simulink model "sim_instalacja_podlogowa_regulacja_pogodowa"  (R2021b)
settings: Solver=VariableStepAuto  StartTime=0.0  StopTime=10.0  MaxStep=10  RelTol=1e-3
undefined symbols (not defined in the file): ap_bojlera, az, az_bojlera, bp_bojlera, bz, bz_bojlera, cpw, Cvcwu, Cvgp, Cvk, Cvp, Cvr, Cvs, Cvw, delay, dpoN, dqt, dqtb, dqtb2, dRz_b, dRz_p, dTcwu, dTzew, fmbN, Kcp1, Kcp2, Kcr, Kcs, Kcw, ki_main, ki_zaw_bojler, ki_zaw_podloga, kp_main, kp_zaw_bojler, kp_zaw_podloga, qtb2N, qtbN, qtN, Rb, Rk, Rp, RzN, skok_czas, skok_czas0, skok_czas2, Tcwu0, TcwuN, Tgp0, TkpN, Tkz0, TkzN, Tp0, Trp0, TrpN, Ts0, Tset_cwu, Twew0, TwewK, Tzadana0, TzewN ... (+1)
libraries: slpidlib x3, simulink x1
settings Model: Creator=adams  LastModifiedBy=adams

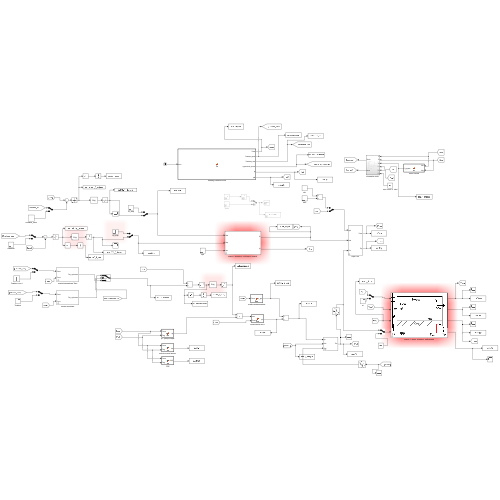
[thumbnail: Simulink's stored preview of the top-level diagram]
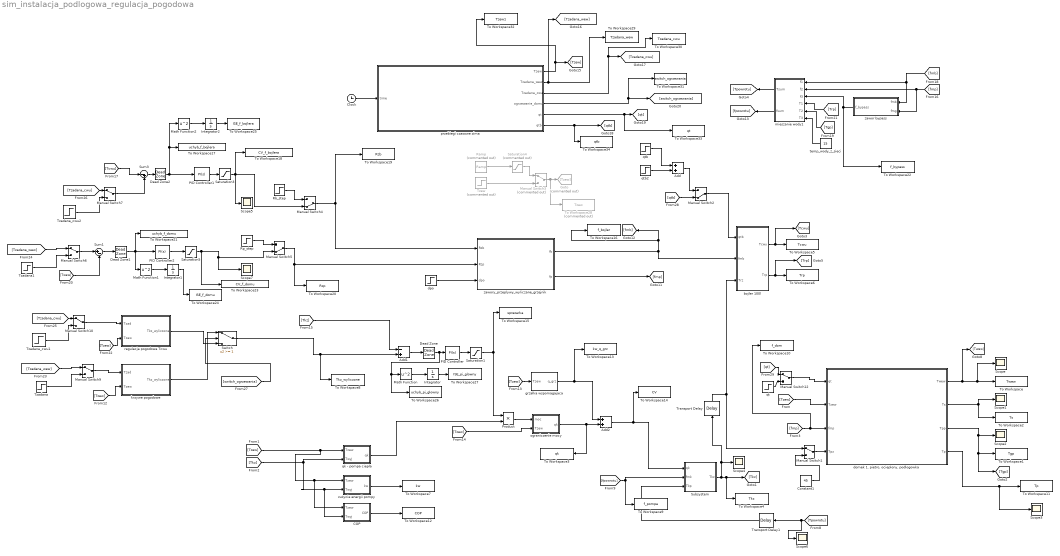
== system sim_instalacja_podlogowa_regulacja_pogodowa ==
  Add : Sum
  Add1 : Sum  Inputs=-+
  Add2 : Sum
  COP : MATLAB Function  TreatAsAtomicUnit=on
  Clock : Clock
  Constant1 : Constant  Value=45
  Dead Zone : DeadZone  LowerValue=-0.15  UpperValue=0.15  SaturateOnIntegerOverflow=on
  Dead Zone1 : DeadZone  LowerValue=-0.55  UpperValue=0.55  SaturateOnIntegerOverflow=on
  Dead Zone2 : DeadZone  LowerValue=-0.35  UpperValue=0.35  SaturateOnIntegerOverflow=on
  Goto : Goto  Commented=on  GotoTag=Tzew
  Integrator : Integrator
  Integrator1 : Integrator
  Integrator2 : Integrator
  Manual Switch{1,6..7,9..10,12} (6 alike) : ManualSwitch
  Manual Switch2 : ManualSwitch  CurrentSetting=0
  Manual Switch3 : ManualSwitch  Commented=on
  Manual Switch4 : ManualSwitch  CurrentSetting=0
  Manual Switch5 : ManualSwitch  CurrentSetting=0
  Math Function : Math  Operator=square  SaturateOnIntegerOverflow=on
  Math Function1 : Math  Operator=square  SaturateOnIntegerOverflow=on
  Math Function2 : Math  Operator=square  SaturateOnIntegerOverflow=on
  PID Controller : slpidlib/PID Controller  Controller=PI  Form=Parallel  TimeDomain=Continuous-time  UseExternalTs=off  SampleTime=-1  IntegratorMethod=Forward Euler  FilterMethod=Forward Euler  ControllerParametersSource=internal  P=kp_main  I=ki_main  D=0  UseFilter=on  N=100  TunerSelectOption=Transfer Function Based (PID Tuner App)  InitialConditionSource=internal  InitialConditionForIntegrator=1  InitialConditionForFilter=0  DifferentiatorICPrevScaledInput=0  ExternalReset=none  TrackingMode=off  Kt=1  LimitOutput=off  SatLimitsSource=internal  UpperSaturationLimit=inf  LowerSaturationLimit=-inf  LinearizeAsGain=on  AntiWindupMode=none  Kb=1  POutMin=[]  POutMax=[]  IOutMin=[]  IOutMax=[]  DOutMin=[]  DOutMax=[]  NOutMin=[]  NOutMax=[]  SumOutMin=[]  SumOutMax=[]  SaturationOutMin=[]  SaturationOutMax=[]  PParamMin=[]  PParamMax=[]  IParamMin=[]  IParamMax=[]  DParamMin=[]  DParamMax=[]  NParamMin=[]  NParamMax=[]  KbParamMin=[]  KbParamMax=[]  KtParamMin=[]  KtParamMax=[]  KbOutMin=[]  KbOutMax=[]  KtOutMin=[]  KtOutMax=[]  IntegratorOutMin=[]  IntegratorOutMax=[]  FilterOutMin=[]  FilterOutMax=[]  SumI1OutMin=[]  SumI1OutMax=[]  SumI2OutMin=[]  SumI2OutMax=[]  SumI3OutMin=[]  SumI3OutMax=[]  SumI4OutMin=[]  SumI4OutMax=[]  SumDOutMin=[]  SumDOutMax=[]  DifferentiatorOutMin=[]  DifferentiatorOutMax=[]  FilterDiffOutCoefMin=[]  FilterDiffOutCoefMax=[]  ReciprocalOutMin=[]  ReciprocalOutMax=[]  SumDenOutMin=[]  SumDenOutMax=[]  SumNumOutMin=[]  SumNumOutMax=[]  DivideOutMin=[]  DivideOutMax=[]  UdiffTsProdOutMin=[]  UdiffTsProdOutMax=[]  NTsProdOutMin=[]  NTsProdOutMax=[]  UintegralTsProdOutMin=[]  UintegralTsProdOutMax=[]  UngainTsProdOutMin=[]  UngainTsProdOutMax=[]  FilterDenConstantOutDataTypeStr=Inherit: Inherit via back propagation  FilterDenConstantOutMin=[]  FilterDenConstantOutMax=[]  PCopyOutDataTypeStr=Inherit: Inherit via back propagation  PCopyOutMin=[]  PCopyOutMax=[]  NCopyOutDataTypeStr=Inherit: Inherit via back propagation  NCopyOutMin=[]  NCopyOutMax=[]  IntegratorContinuousStateAttributes=''  IntegratorStateMustResolveToSignalObject=off  IntegratorRTWStateStorageClass=Auto  FilterContinuousStateAttributes=''  FilterStateMustResolveToSignalObject=off  FilterRTWStateStorageClass=Auto  ParallelPVariant=InternalParameters  IdealPVariant=Disabled  IVariant=InternalParameters  DVariant=Disabled  IntegratorVariant=Continuous  SatVariant=Disabled  AWVariant=Passthrough  PCopyVariant=Disabled  TRVariant=Disabled  FdbkBlocksVariant=Forward  IdealPFdbkVariant=Disabled  SatFdbkVariant=Disabled  DerivativeFilterVariant=Disabled  NVariant=Disabled  NCopyVariant=Disabled_SignalSpec  FilterICVariant=Disabled  IntegratorICVariant=InternalICs  ExternalResetVariant=Disabled  TRSumVariant=Passthrough  SumFdbkVariant=Disabled  SumVariant=Sum_PI  TsampFilterVariant=InternalTs  TsampNgainVariant=Passthrough  TsampIntegralVariant=Passthrough  ExternalSaturationOutDataTypeStr=Inherit: Same as second input
  PID Controller1 : slpidlib/PID Controller  Controller=PI  Form=Parallel  TimeDomain=Continuous-time  UseExternalTs=off  SampleTime=-1  IntegratorMethod=Forward Euler  FilterMethod=Forward Euler  ControllerParametersSource=internal  P=kp_zaw_bojler  I=ki_zaw_bojler  D=0  UseFilter=on  N=100  TunerSelectOption=Transfer Function Based (PID Tuner App)  InitialConditionSource=internal  InitialConditionForIntegrator=0  InitialConditionForFilter=0  DifferentiatorICPrevScaledInput=0  ExternalReset=none  TrackingMode=off  Kt=1  LimitOutput=off  SatLimitsSource=internal  UpperSaturationLimit=inf  LowerSaturationLimit=-inf  LinearizeAsGain=on  AntiWindupMode=none  Kb=1  POutMin=[]  POutMax=[]  IOutMin=[]  IOutMax=[]  DOutMin=[]  DOutMax=[]  NOutMin=[]  NOutMax=[]  SumOutMin=[]  SumOutMax=[]  SaturationOutMin=[]  SaturationOutMax=[]  PParamMin=[]  PParamMax=[]  IParamMin=[]  IParamMax=[]  DParamMin=[]  DParamMax=[]  NParamMin=[]  NParamMax=[]  KbParamMin=[]  KbParamMax=[]  KtParamMin=[]  KtParamMax=[]  KbOutMin=[]  KbOutMax=[]  KtOutMin=[]  KtOutMax=[]  IntegratorOutMin=[]  IntegratorOutMax=[]  FilterOutMin=[]  FilterOutMax=[]  SumI1OutMin=[]  SumI1OutMax=[]  SumI2OutMin=[]  SumI2OutMax=[]  SumI3OutMin=[]  SumI3OutMax=[]  SumI4OutMin=[]  SumI4OutMax=[]  SumDOutMin=[]  SumDOutMax=[]  DifferentiatorOutMin=[]  DifferentiatorOutMax=[]  FilterDiffOutCoefMin=[]  FilterDiffOutCoefMax=[]  ReciprocalOutMin=[]  ReciprocalOutMax=[]  SumDenOutMin=[]  SumDenOutMax=[]  SumNumOutMin=[]  SumNumOutMax=[]  DivideOutMin=[]  DivideOutMax=[]  UdiffTsProdOutMin=[]  UdiffTsProdOutMax=[]  NTsProdOutMin=[]  NTsProdOutMax=[]  UintegralTsProdOutMin=[]  UintegralTsProdOutMax=[]  UngainTsProdOutMin=[]  UngainTsProdOutMax=[]  FilterDenConstantOutDataTypeStr=Inherit: Inherit via back propagation  FilterDenConstantOutMin=[]  FilterDenConstantOutMax=[]  PCopyOutDataTypeStr=Inherit: Inherit via back propagation  PCopyOutMin=[]  PCopyOutMax=[]  NCopyOutDataTypeStr=Inherit: Inherit via back propagation  NCopyOutMin=[]  NCopyOutMax=[]  IntegratorContinuousStateAttributes=''  IntegratorStateMustResolveToSignalObject=off  IntegratorRTWStateStorageClass=Auto  FilterContinuousStateAttributes=''  FilterStateMustResolveToSignalObject=off  FilterRTWStateStorageClass=Auto  ParallelPVariant=InternalParameters  IdealPVariant=Disabled  IVariant=InternalParameters  DVariant=Disabled  IntegratorVariant=Continuous  SatVariant=Disabled  AWVariant=Passthrough  PCopyVariant=Disabled  TRVariant=Disabled  FdbkBlocksVariant=Forward  IdealPFdbkVariant=Disabled  SatFdbkVariant=Disabled  DerivativeFilterVariant=Disabled  NVariant=Disabled  NCopyVariant=Disabled_SignalSpec  FilterICVariant=Disabled  IntegratorICVariant=InternalICs  ExternalResetVariant=Disabled  TRSumVariant=Passthrough  SumFdbkVariant=Disabled  SumVariant=Sum_PI  TsampFilterVariant=InternalTs  TsampNgainVariant=Passthrough  TsampIntegralVariant=Passthrough  ExternalSaturationOutDataTypeStr=Inherit: Same as second input
  PID Controller2 : slpidlib/PID Controller  Controller=PI  Form=Parallel  TimeDomain=Continuous-time  UseExternalTs=off  SampleTime=-1  IntegratorMethod=Forward Euler  FilterMethod=Forward Euler  ControllerParametersSource=internal  P=kp_zaw_podloga  I=ki_zaw_podloga  D=0  UseFilter=on  N=100  TunerSelectOption=Transfer Function Based (PID Tuner App)  InitialConditionSource=internal  InitialConditionForIntegrator=0  InitialConditionForFilter=0  DifferentiatorICPrevScaledInput=0  ExternalReset=none  TrackingMode=off  Kt=1  LimitOutput=off  SatLimitsSource=internal  UpperSaturationLimit=inf  LowerSaturationLimit=-inf  LinearizeAsGain=on  AntiWindupMode=none  Kb=1  POutMin=[]  POutMax=[]  IOutMin=[]  IOutMax=[]  DOutMin=[]  DOutMax=[]  NOutMin=[]  NOutMax=[]  SumOutMin=[]  SumOutMax=[]  SaturationOutMin=[]  SaturationOutMax=[]  PParamMin=[]  PParamMax=[]  IParamMin=[]  IParamMax=[]  DParamMin=[]  DParamMax=[]  NParamMin=[]  NParamMax=[]  KbParamMin=[]  KbParamMax=[]  KtParamMin=[]  KtParamMax=[]  KbOutMin=[]  KbOutMax=[]  KtOutMin=[]  KtOutMax=[]  IntegratorOutMin=[]  IntegratorOutMax=[]  FilterOutMin=[]  FilterOutMax=[]  SumI1OutMin=[]  SumI1OutMax=[]  SumI2OutMin=[]  SumI2OutMax=[]  SumI3OutMin=[]  SumI3OutMax=[]  SumI4OutMin=[]  SumI4OutMax=[]  SumDOutMin=[]  SumDOutMax=[]  DifferentiatorOutMin=[]  DifferentiatorOutMax=[]  FilterDiffOutCoefMin=[]  FilterDiffOutCoefMax=[]  ReciprocalOutMin=[]  ReciprocalOutMax=[]  SumDenOutMin=[]  SumDenOutMax=[]  SumNumOutMin=[]  SumNumOutMax=[]  DivideOutMin=[]  DivideOutMax=[]  UdiffTsProdOutMin=[]  UdiffTsProdOutMax=[]  NTsProdOutMin=[]  NTsProdOutMax=[]  UintegralTsProdOutMin=[]  UintegralTsProdOutMax=[]  UngainTsProdOutMin=[]  UngainTsProdOutMax=[]  FilterDenConstantOutDataTypeStr=Inherit: Inherit via back propagation  FilterDenConstantOutMin=[]  FilterDenConstantOutMax=[]  PCopyOutDataTypeStr=Inherit: Inherit via back propagation  PCopyOutMin=[]  PCopyOutMax=[]  NCopyOutDataTypeStr=Inherit: Inherit via back propagation  NCopyOutMin=[]  NCopyOutMax=[]  IntegratorContinuousStateAttributes=''  IntegratorStateMustResolveToSignalObject=off  IntegratorRTWStateStorageClass=Auto  FilterContinuousStateAttributes=''  FilterStateMustResolveToSignalObject=off  FilterRTWStateStorageClass=Auto  ParallelPVariant=InternalParameters  IdealPVariant=Disabled  IVariant=InternalParameters  DVariant=Disabled  IntegratorVariant=Continuous  SatVariant=Disabled  AWVariant=Passthrough  PCopyVariant=Disabled  TRVariant=Disabled  FdbkBlocksVariant=Forward  IdealPFdbkVariant=Disabled  SatFdbkVariant=Disabled  DerivativeFilterVariant=Disabled  NVariant=Disabled  NCopyVariant=Disabled_SignalSpec  FilterICVariant=Disabled  IntegratorICVariant=InternalICs  ExternalResetVariant=Disabled  TRSumVariant=Passthrough  SumFdbkVariant=Disabled  SumVariant=Sum_PI  TsampFilterVariant=InternalTs  TsampNgainVariant=Passthrough  TsampIntegralVariant=Passthrough  ExternalSaturationOutDataTypeStr=Inherit: Same as second input
  Product : Product
  Ramp : simulink/Sources/Ramp  Commented=on  slope=0.00003091  start=skok_czas0  InitialOutput=TzewN
  Rb_step : Step  Time=skok_czas2  Before=RzN  After=RzN + dRz_b  SampleTime=0
  Rp_step : Step  Time=skok_czas2  Before=RzN  After=RzN + dRz_p  SampleTime=0
  Saturation1 : Saturate  UpperLimit=1.42  LowerLimit=0.1
  Saturation3 : Saturate  UpperLimit=999999999999999999999999999999999999999999  LowerLimit=0
  Saturation4 : Saturate  Commented=on  UpperLimit=-4  LowerLimit=-10
  Saturation5 : Saturate  UpperLimit=999999999999999999999999999999999999999999  LowerLimit=0
  Scope{,1..7} (8 alike) : Scope
  Subsystem : Subsystem  mask{Cvk=Cvk, cpw=cpw, Tkz0=Tkz0}
  Sum1 : Sum  Inputs=|+-
  Sum3 : Sum  Inputs=|-+
  Switch : Switch  Threshold=1
  To Workspace : ToWorkspace  VariableName=Twew  SampleTime=-1
  To Workspace1 : ToWorkspace  VariableName=Tgp  SampleTime=-1
  To Workspace10 : ToWorkspace  VariableName=f_dom  SampleTime=-1
  To Workspace11 : ToWorkspace  VariableName=Tp  SampleTime=-1
  To Workspace12 : ToWorkspace  VariableName=COP  SampleTime=-1
  To Workspace13 : ToWorkspace  VariableName=kw_q_grz  SampleTime=-1
  To Workspace14 : ToWorkspace  VariableName=CV  SampleTime=-1
  To Workspace15 : ToWorkspace  VariableName=sprezarka  SampleTime=-1
  To Workspace16 : ToWorkspace  VariableName=f_bojler  SampleTime=-1
  To Workspace17 : ToWorkspace  VariableName=uchyb_f_bojlera  SampleTime=-1
  To Workspace18 : ToWorkspace  VariableName=CV_f_bojlera  SampleTime=-1
  To Workspace19 : ToWorkspace  VariableName=Rzb  SampleTime=-1
  To Workspace2 : ToWorkspace  VariableName=Ts  SampleTime=-1
  To Workspace20 : ToWorkspace  VariableName=Rzp  SampleTime=-1
  To Workspace21 : ToWorkspace  VariableName=uchyb_f_domu  SampleTime=-1
  To Workspace22 : ToWorkspace  VariableName=f_bypass  SampleTime=-1
  To Workspace23 : ToWorkspace  VariableName=CV_f_domu  SampleTime=-1
  To Workspace24 : ToWorkspace  VariableName=ISE_f_domu  SampleTime=-1
  To Workspace25 : ToWorkspace  VariableName=ISE_f_bojlera  SampleTime=-1
  To Workspace26 : ToWorkspace  VariableName=uchyb_pi_glowny  SampleTime=-1
  To Workspace27 : ToWorkspace  VariableName=ISE_pi_glowny  SampleTime=-1
  To Workspace28 : ToWorkspace  Commented=on  VariableName=Tzew  SampleTime=-1
  To Workspace29 : ToWorkspace  VariableName=Tzadana_wew  SampleTime=-1
  To Workspace3 : ToWorkspace  VariableName=qk  SampleTime=-1
  To Workspace30 : ToWorkspace  VariableName=Tzadana_cwu  SampleTime=-1
  To Workspace31 : ToWorkspace  VariableName=switch_ogrzewania  SampleTime=-1
  To Workspace32 : ToWorkspace  VariableName=Tzew1  SampleTime=-1
  To Workspace33 : ToWorkspace  VariableName=qt  SampleTime=-1
  To Workspace34 : ToWorkspace  VariableName=qtb  SampleTime=-1
  To Workspace4 : ToWorkspace  VariableName=Tkz  SampleTime=-1
  To Workspace5 : ToWorkspace  VariableName=Tcwu  SampleTime=-1
  To Workspace6 : ToWorkspace  VariableName=Trp  SampleTime=-1
  To Workspace7 : ToWorkspace  VariableName=kw  SampleTime=-1
  To Workspace8 : ToWorkspace  VariableName=Tkz_wyliczone  SampleTime=-1
  To Workspace9 : ToWorkspace  VariableName=f_pompa  SampleTime=-1
  Transport Delay : TransportDelay  DelayTime=delay  InitialOutput=TkzN
  Transport Delay1 : TransportDelay  DelayTime=delay  InitialOutput=TkpN
  Tzadana : Step  Time=skok_czas  Before=Tzadana0  After=TwewK  SampleTime=0
  Tzadana1 : Step  Time=skok_czas  Before=Tzadana0  After=TwewK  SampleTime=0
  Tzadana_cwu1 : Step  Time=skok_czas  Before=Tset_cwu  After="Tset_cwu  + dTcwu"  SampleTime=0
  Tzadana_cwu2 : Step  Time=skok_czas  Before=Tset_cwu  After="Tset_cwu  + dTcwu"  SampleTime=0
  Tzew : Step  Commented=on  Time=skok_czas0  Before=TzewN  After=TzewN+dTzew  SampleTime=0
  bojler 100l : Subsystem  mask{Kcr=Kcr, cpw=cpw, Cvr=Cvr, Cvcwu=Cvcwu, TcwuN=TcwuN, TrpN=TrpN}
  "domek 1. pietro, ocieplony, podlogowka" : Subsystem  mask{Tp0=Tp0, Tgp0=Tgp0, Twew0=Twew0, Ts0=Ts0, cpw=cpw, Kcs=Kcs, Kcw=Kcw, Kcp1=Kcp1, Kcp2=Kcp2, Cvp=Cvp, Cvgp=Cvgp, Cvs=Cvs, Cvw=Cvw}
      mask Display: image('D:\Dokumenty\Studia\7. sem\schemat podlogowki.png'); % Use "Edit Image" on toolstrip to change.
  dpo : Step  Time=skok_czas  Before=dpoN  After=dpoN + zmiana_po  SampleTime=0
  grzałka wspomagajaca : MATLAB Function  TreatAsAtomicUnit=on
  krzywe pogodowe : Subsystem  mask{az=az, bz=bz}
  mieszanie wody1 : Subsystem
  ograniczenie mocy : MATLAB Function  TreatAsAtomicUnit=on
  przebiegi czasowe zima : MATLAB Function  TreatAsAtomicUnit=on
  qk - pompa ciepła : MATLAB Function  TreatAsAtomicUnit=on
  qt : Step  Time=skok_czas  Before=qtN  After=qtN+dqt  SampleTime=0
  qtb : Step  Time=skok_czas  Before=qtbN  After=qtbN + dqtb  SampleTime=0
  qtb2 : Step  Time=skok_czas2  Before=qtb2N  After=qtb2N + dqtb2  SampleTime=0  ZeroCross=off
  regulacja pogodowa Tcwu : Subsystem  mask{az=az_bojlera, bz=bz_bojlera, ap=ap_bojlera, bp=bp_bojlera, cpw=cpw, fmgN=fmbN}
  temp_wody_z_sieci : Constant  Value=15
  zawor bypass : MATLAB Function  TreatAsAtomicUnit=on
  zawory_przeplywy_wyliczane_grzejnik : Subsystem  mask{Rk=Rk, Rb=Rb, Rp=Rp}
  zużycie energii pompy : MATLAB Function  TreatAsAtomicUnit=on
  wires:
  [Tkz] -> qk - pompa ciepła/2(Twyj), COP/2(Twyj), zużycie energii pompy/2(Twyj)
  ograniczenie mocy/1(qk) -> To Workspace3/1, Add2/2
  grzałka wspomagajaca/1(q_grz) -> To Workspace13/1, Add2/1
  Add2/1 -> To Workspace14/1, Subsystem/1(qk)
  bojler 100l/1(Tcwu) -> [Tcwu], To Workspace5/1
  [Tzew] -> grzałka wspomagajaca/1(Tzew)
  Product/1 -> ograniczenie mocy/1(moc)
  bojler 100l/2(Trp) -> [Trp], To Workspace6/1
  [Tzew] -> krzywe pogodowe/2(Tzew)
  qk - pompa ciepła/1(qk) -> Product/2
  [fpowrotu] -> Subsystem/2(fmk), To Workspace9/1
  [Tzew] -> ograniczenie mocy/2(Tzew)
  "domek 1. pietro, ocieplony, podlogowka"/2(Ts) -> To Workspace2/1, Scope1/1
  "domek 1. pietro, ocieplony, podlogowka"/1(Twew) -> [Twew], Scope/1, To Workspace/1
  "domek 1. pietro, ocieplony, podlogowka"/3(Tpp) -> To Workspace1/1, [Tgp], Scope2/1
  Subsystem/1(Tkz) -> Scope4/1, Transport Delay/1, [Tkz], To Workspace4/1
  zużycie energii pompy/1(kw) -> To Workspace7/1
  Transport Delay/1 -> Manual Switch1/1, bojler 100l/3(Trz)
  COP/1(COP) -> To Workspace12/1
  [Tpowrotu] -> Scope6/1, Transport Delay1/1
  [Tzew] -> "domek 1. pietro, ocieplony, podlogowka"/2(Tzew)
  Saturation1/1 -> To Workspace15/1, Product/1
  Transport Delay1/1 -> Subsystem/3(Tkp)
  Manual Switch5/1 -> zawory_przeplywy_wyliczane_grzejnik/2(Rzp), To Workspace20/1
  [fmp] -> To Workspace10/1, "domek 1. pietro, ocieplony, podlogowka"/3(fmp)
  [Tzew] -> qk - pompa ciepła/1(Tzew), zużycie energii pompy/1(Tzew), COP/1(Tzew)
  Manual Switch4/1 -> To Workspace19/1, zawory_przeplywy_wyliczane_grzejnik/1(Rzb)
  zawory_przeplywy_wyliczane_grzejnik/1(fb) -> bojler 100l/2(fmb), To Workspace16/1, [fmb]
  dpo/1 -> zawory_przeplywy_wyliczane_grzejnik/3(dpo)
  "domek 1. pietro, ocieplony, podlogowka"/4(Tp) -> To Workspace11/1, Scope3/1
  zawory_przeplywy_wyliczane_grzejnik/2(fp) -> [fmp]
  [Tkz] -> Add1/1
  PID Controller/1 -> Saturation1/1
  Add1/1 -> Dead Zone/1
  Constant1/1 -> Manual Switch1/2
  Manual Switch1/1 -> "domek 1. pietro, ocieplony, podlogowka"/4(Tpz)
  [Tgp] -> mieszanie wody1/5(T2)
  [fmb] -> mieszanie wody1/1(f1), zawor bypass/1(fmb)
  zawor bypass/1(f_bypass) -> mieszanie wody1/3(f3), To Workspace22/1
  mieszanie wody1/2(fsum) -> [fpowrotu]
  mieszanie wody1/1(Tsum) -> [Tpowrotu]
  [Trp] -> mieszanie wody1/4(T1)
  temp_wody_z_sieci/1 -> mieszanie wody1/6(T3)
  [fmp] -> zawor bypass/2(fmg), mieszanie wody1/2(f2)
  PID Controller2/1 -> Saturation5/1
  Dead Zone1/1 -> Math Function1/1, To Workspace21/1, PID Controller2/1
  [Tcwu] -> Sum3/1
  [Twew] -> Sum1/2
  Sum3/1 -> Dead Zone2/1
  Sum1/1 -> Dead Zone1/1
  PID Controller1/1 -> Saturation3/1
  Rp_step/1 -> Manual Switch5/1
  Saturation5/1 -> To Workspace23/1, Scope7/1, Manual Switch5/2
  Rb_step/1 -> Manual Switch4/1
  Saturation3/1 -> Manual Switch4/2, To Workspace18/1, Scope5/1
  Integrator2/1 -> To Workspace25/1
  Dead Zone2/1 -> Math Function2/1, To Workspace17/1, PID Controller1/1
  Math Function2/1 -> Integrator2/1
  Math Function1/1 -> Integrator1/1
  Integrator1/1 -> To Workspace24/1
  Dead Zone/1 -> To Workspace26/1, Math Function/1, PID Controller/1
  Integrator/1 -> To Workspace27/1
  Math Function/1 -> Integrator/1
  Manual Switch3/1 -> To Workspace28/1, Goto/1
  Tzew/1 -> Manual Switch3/2
  Ramp/1 -> Saturation4/1
  Saturation4/1 -> Manual Switch3/1
  Manual Switch10/1 -> regulacja pogodowa Tcwu/1(Tzad)
  [Tzew] -> regulacja pogodowa Tcwu/2(Tzew)
  regulacja pogodowa Tcwu/1(Tkz_wyliczone) -> Switch/3
  krzywe pogodowe/1(Tkz_wyliczone) -> Switch/1
  Switch/1 -> To Workspace8/1, Add1/2
  Manual Switch9/1 -> krzywe pogodowe/1(Tzad)
  Tzadana/1 -> Manual Switch9/2
  [Tzadana_wew] -> Manual Switch9/1
  Manual Switch6/1 -> Sum1/1
  Tzadana1/1 -> Manual Switch6/2
  [Tzadana_wew] -> Manual Switch6/1
  [Tzadana_cwu] -> Manual Switch10/1
  Tzadana_cwu1/1 -> Manual Switch10/2
  [Tzadana_cwu] -> Manual Switch7/1
  Tzadana_cwu2/1 -> Manual Switch7/2
  Manual Switch7/1 -> Sum3/2
  [switch_ogrzewania] -> Switch/2
  qtb2/1 -> Add/2
  [qtb] -> Manual Switch2/2
  Add/1 -> Manual Switch2/1
  Manual Switch2/1 -> bojler 100l/1(qtb)
  qtb/1 -> Add/1
  Manual Switch12/1 -> "domek 1. pietro, ocieplony, podlogowka"/1(qt)
  [qt] -> Manual Switch12/1
  qt/1 -> Manual Switch12/2
  Clock/1 -> przebiegi czasowe zima/1(time)
  przebiegi czasowe zima/5(qt) -> To Workspace33/1, [qt]
  przebiegi czasowe zima/6(qtb) -> To Workspace34/1, [qtb]
  przebiegi czasowe zima/3(Tzadana_cwu) -> To Workspace30/1, [Tzadana_cwu]
  przebiegi czasowe zima/4(ogrzewanie_domu) -> [switch_ogrzewania], To Workspace31/1
  przebiegi czasowe zima/1(Tzew) -> To Workspace32/1, [Tzew]
  przebiegi czasowe zima/2(Tzadana_wew) -> To Workspace29/1, [Tzadana_wew]

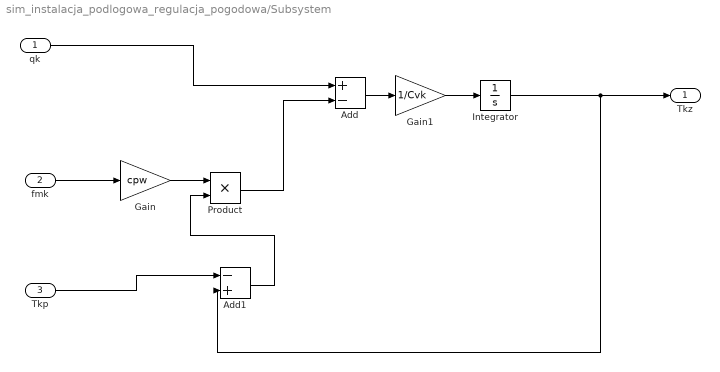
== system sim_instalacja_podlogowa_regulacja_pogodowa/Subsystem ==
  qk : Inport
  fmk : Inport  Port=2
  Tkp : Inport  Port=3
  Add : Sum  Inputs=+-
  Add1 : Sum  Inputs=-+
  Gain : Gain  Gain=cpw
  Gain1 : Gain  Gain=1/Cvk
  Integrator : Integrator  InitialCondition=Tkz0
  Product : Product
  Tkz : Outport
  wires:
  Add1/1 -> Product/2
  Gain/1 -> Product/1
  Integrator/1 -> Add1/2, Tkz/1
  Add/1 -> Gain1/1
  Tkp/1 -> Add1/1
  Gain1/1 -> Integrator/1
  Product/1 -> Add/2
  fmk/1 -> Gain/1
  qk/1 -> Add/1

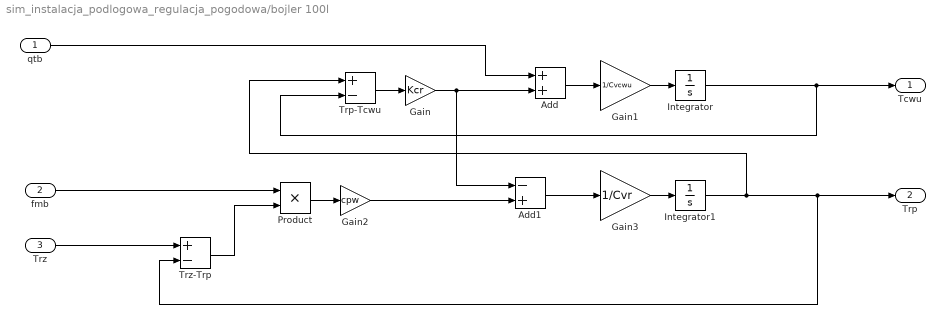
== system sim_instalacja_podlogowa_regulacja_pogodowa/bojler 100l ==
  qtb : Inport
  fmb : Inport  Port=2
  Trz : Inport  Port=3
  Add : Sum
  Add1 : Sum  Inputs=-+
  Gain : Gain  Gain=Kcr
  Gain1 : Gain  Gain=1/Cvcwu
  Gain2 : Gain  Gain=cpw
  Gain3 : Gain  Gain=1/Cvr
  Integrator : Integrator  InitialCondition=Tcwu0
  Integrator1 : Integrator  InitialCondition=Trp0
  Product : Product
  Trp-Tcwu : Sum  Inputs=+-
  Trz-Trp : Sum  Inputs=+-
  Tcwu : Outport
  Trp : Outport  Port=2
  wires:
  Gain/1 -> Add/2, Add1/1
  Add/1 -> Gain1/1
  Trz-Trp/1 -> Product/2
  fmb/1 -> Product/1
  Product/1 -> Gain2/1
  Gain1/1 -> Integrator/1
  Trp-Tcwu/1 -> Gain/1
  Gain3/1 -> Integrator1/1
  Integrator/1 -> Tcwu/1, Trp-Tcwu/2
  Gain2/1 -> Add1/2
  Add1/1 -> Gain3/1
  Integrator1/1 -> Trp-Tcwu/1, Trp/1, Trz-Trp/2
  Trz/1 -> Trz-Trp/1
  qtb/1 -> Add/1

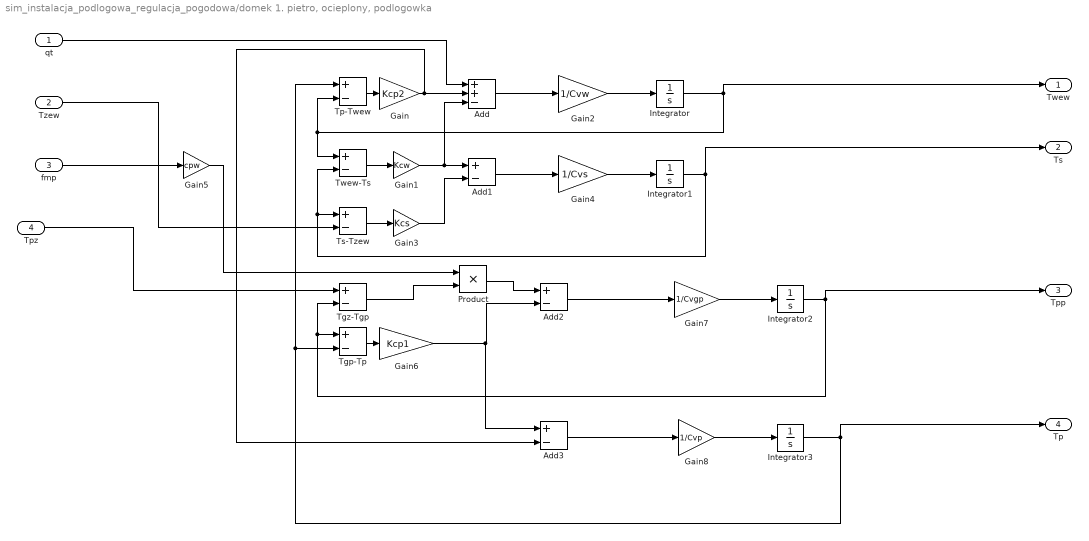
== system sim_instalacja_podlogowa_regulacja_pogodowa/domek 1. pietro, ocieplony, podlogowka ==
  qt : Inport
  Tzew : Inport  Port=2
  fmp : Inport  Port=3
  Tpz : Inport  Port=4
  Add : Sum  Inputs=++-
  Add1 : Sum  Inputs=+-
  Add2 : Sum  Inputs=+-
  Add3 : Sum  Inputs=+-
  Gain : Gain  Gain=Kcp2
  Gain1 : Gain  Gain=Kcw
  Gain2 : Gain  Gain=1/Cvw
  Gain3 : Gain  Gain=Kcs
  Gain4 : Gain  Gain=1/Cvs
  Gain5 : Gain  Gain=cpw
  Gain6 : Gain  Gain=Kcp1
  Gain7 : Gain  Gain=1/Cvgp
  Gain8 : Gain  Gain=1/Cvp
  Integrator : Integrator  InitialCondition=Twew0
  Integrator1 : Integrator  InitialCondition=Ts0
  Integrator2 : Integrator  InitialCondition=Tgp0
  Integrator3 : Integrator  InitialCondition=Tp0
  Product : Product
  Tgp-Tp : Sum  Inputs=+-
  Tgz-Tgp : Sum  Inputs=+-
  Tp-Twew : Sum  Inputs=+-
  Ts-Tzew : Sum  Inputs=+-
  Twew-Ts : Sum  Inputs=+-
  Twew : Outport
  Ts : Outport  Port=2
  Tpp : Outport  Port=3
  Tp : Outport  Port=4
  wires:
  Integrator/1 -> Twew/1, Tp-Twew/2, Twew-Ts/1
  Gain/1 -> Add/2, Add3/2
  Gain6/1 -> Add3/1, Add2/2
  Twew-Ts/1 -> Gain1/1
  Integrator1/1 -> Ts/1, Twew-Ts/2, Ts-Tzew/1
  Gain3/1 -> Add1/2
  Add/1 -> Gain2/1
  Gain2/1 -> Integrator/1
  Tgp-Tp/1 -> Gain6/1
  Gain1/1 -> Add1/1, Add/3
  Product/1 -> Add2/1
  Add1/1 -> Gain4/1
  Ts-Tzew/1 -> Gain3/1
  Gain5/1 -> Product/1
  Add3/1 -> Gain8/1
  qt/1 -> Add/1
  Integrator2/1 -> Tpp/1, Tgp-Tp/1, Tgz-Tgp/2
  Tgz-Tgp/1 -> Product/2
  Gain7/1 -> Integrator2/1
  Tp-Twew/1 -> Gain/1
  Integrator3/1 -> Tp/1, Tp-Twew/1, Tgp-Tp/2
  Gain8/1 -> Integrator3/1
  Gain4/1 -> Integrator1/1
  Add2/1 -> Gain7/1
  Tzew/1 -> Ts-Tzew/2
  fmp/1 -> Gain5/1
  Tpz/1 -> Tgz-Tgp/1

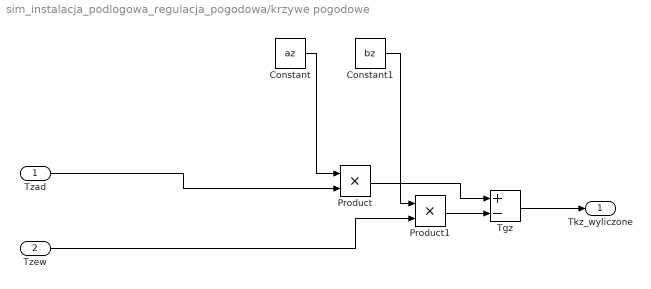
== system sim_instalacja_podlogowa_regulacja_pogodowa/krzywe pogodowe ==
  Tzad : Inport
  Tzew : Inport  Port=2
  Constant : Constant  Value=az
  Constant1 : Constant  Value=bz
  Product : Product
  Product1 : Product
  Tgz : Sum  Inputs=+-
  Tkz_wyliczone : Outport
  wires:
  Product/1 -> Tgz/1
  Constant1/1 -> Product1/1
  Product1/1 -> Tgz/2
  Tzad/1 -> Product/2
  Tgz/1 -> Tkz_wyliczone/1
  Tzew/1 -> Product1/2
  Constant/1 -> Product/1

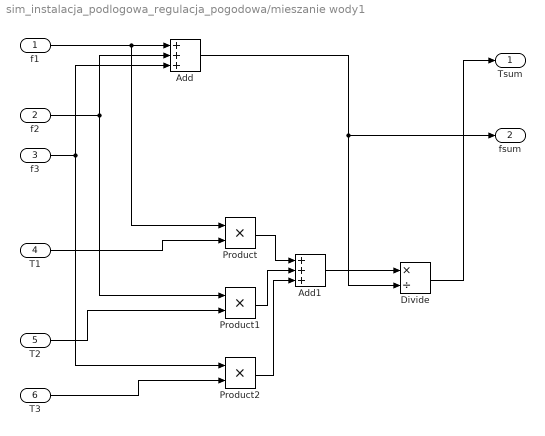
== system sim_instalacja_podlogowa_regulacja_pogodowa/mieszanie wody1 ==
  f1 : Inport
  f2 : Inport  Port=2
  f3 : Inport  Port=3
  T1 : Inport  Port=4
  T2 : Inport  Port=5
  T3 : Inport  Port=6
  Add : Sum  Inputs=+++
  Add1 : Sum  Inputs=+++
  Divide : Product  Inputs=*/
  Product : Product
  Product1 : Product
  Product2 : Product
  Tsum : Outport
  fsum : Outport  Port=2
  wires:
  f2/1 -> Add/2, Product1/1
  f1/1 -> Product/1, Add/1
  Add/1 -> fsum/1, Divide/2
  Product1/1 -> Add1/2
  T2/1 -> Product1/2
  Product/1 -> Add1/1
  Add1/1 -> Divide/1
  T1/1 -> Product/2
  Divide/1 -> Tsum/1
  f3/1 -> Add/3, Product2/1
  T3/1 -> Product2/2
  Product2/1 -> Add1/3

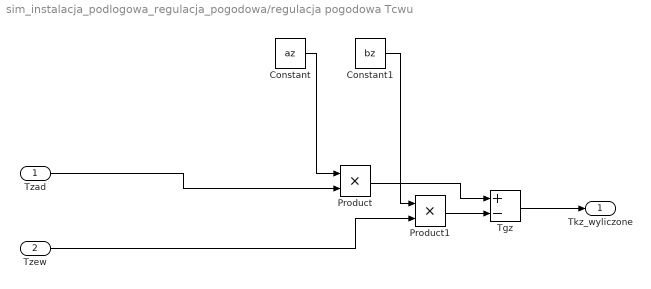
== system sim_instalacja_podlogowa_regulacja_pogodowa/regulacja pogodowa Tcwu ==
  Tzad : Inport
  Tzew : Inport  Port=2
  Constant : Constant  Value=az
  Constant1 : Constant  Value=bz
  Product : Product
  Product1 : Product
  Tgz : Sum  Inputs=+-
  Tkz_wyliczone : Outport
  wires:
  Product/1 -> Tgz/1
  Constant1/1 -> Product1/1
  Product1/1 -> Tgz/2
  Tzad/1 -> Product/2
  Tgz/1 -> Tkz_wyliczone/1
  Tzew/1 -> Product1/2
  Constant/1 -> Product/1

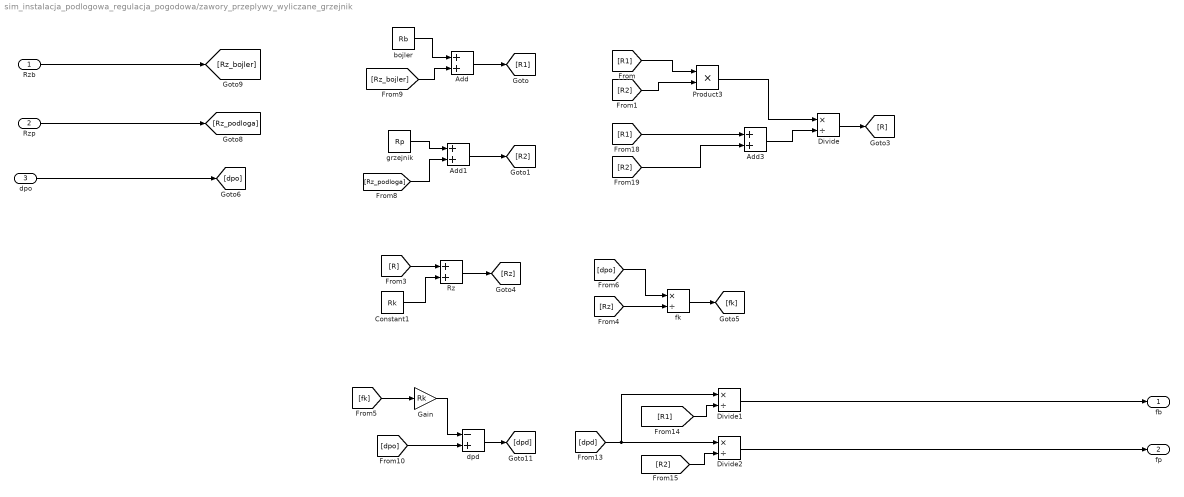
== system sim_instalacja_podlogowa_regulacja_pogodowa/zawory_przeplywy_wyliczane_grzejnik ==
  Rzb : Inport
  Rzp : Inport  Port=2
  dpo : Inport  Port=3
  Add : Sum
  Add1 : Sum
  Add3 : Sum
  Constant1 : Constant  Value=Rk
  Divide : Product  Inputs=*/
  Divide1 : Product  Inputs=*/
  Divide2 : Product  Inputs=*/
  Gain : Gain  Gain=Rk
  Product3 : Product
  Rz : Sum
  bojler : Constant  Value=Rb
  dpd : Sum  Inputs=-+
  fk : Product  Inputs=*/
  grzejnik : Constant  Value=Rp
  fb : Outport
  fp : Outport  Port=2
  wires:
  Divide2/1 -> fp/1
  [R1] -> Add3/1
  [fk] -> Gain/1
  grzejnik/1 -> Add1/1
  Product3/1 -> Divide/1
  bojler/1 -> Add/1
  [R] -> Rz/1
  [R2] -> Add3/2
  Add3/1 -> Divide/2
  [R2] -> Product3/2
  [dpo] -> fk/1
  fk/1 -> [fk]
  [dpd] -> Divide2/1, Divide1/1
  [Rz_bojler] -> Add/2
  Add1/1 -> [R2]
  [R1] -> Divide1/2
  [R1] -> Product3/1
  Divide1/1 -> fb/1
  Constant1/1 -> Rz/2
  [R2] -> Divide2/2
  [Rz_podloga] -> Add1/2
  [dpo] -> dpd/2
  Rzp/1 -> [Rz_podloga]
  Gain/1 -> dpd/1
  Divide/1 -> [R]
  dpd/1 -> [dpd]
  Add/1 -> [R1]
  [Rz] -> fk/2
  Rz/1 -> [Rz]
  dpo/1 -> [dpo]
  Rzb/1 -> [Rz_bojler]

== matlab function sim_instalacja_podlogowa_regulacja_pogodowa/zużycie energii pompy ==
  data: Tzew input; kw output; Twyj input
function kw = fcn(Tzew, Twyj)
kw = 0;
if Twyj >= 50
    if -15 <=Tzew && Tzew < -7
        kw = 35*Tzew + 4235;
    elseif -7 <=Tzew && Tzew < 2
        kw = -20/9*Tzew + 35770/9;
    elseif 2 <=Tzew && Tzew < 7
        kw = -72*Tzew + 4114;
    elseif 7 <=Tzew && Tzew < 10
        kw = -80*Tzew + 4170;
    elseif 10 <=Tzew && Tzew < 20
        kw = 6*Tzew + 3310;
    elseif 20 <=Tzew && Tzew <= 30
        kw = -60*Tzew + 4630;
    else
         fprintf('Error: Tzew out of range [-15;30]\n'); 
    end
elseif Twyj >= 40 && Twyj < 50
%     if -20 <=Tzew && Tzew < -15
%         kw = 54*Tzew + 4020;
%     elseif -15 <=Tzew && Tzew < -7
    if -15 <=Tzew && Tzew < -7
        kw = -25*Tzew + 2835;
    elseif -7 <=Tzew && Tzew < 2
        kw = -530/9*Tzew + 23380/9;
    elseif 2 <=Tzew && Tzew < 10
        kw = 2480;
    elseif 10 <=Tzew && Tzew < 20
        kw = -32*Tzew + 2800;
    elseif 20 <=Tzew && Tzew <= 30
        kw = -49*Tzew + 3100;
    else
%         fprintf('Error: Tzew out of range [-20;30]\n'); 
        fprintf('Error: Tzew out of range [-15;30]\n'); 
    end
elseif Twyj < 40
%         if -20 <=Tzew && Tzew < -15
%             kw = 42*Tzew + 3460;
%         elseif -15 <=Tzew && Tzew < -7
    if -15 <=Tzew && Tzew < -7
        kw = -305/4*Tzew + 6745/4;
    elseif -7 <=Tzew && Tzew < 2
        kw = -550/9*Tzew + 16130/9;
    elseif 2 <=Tzew && Tzew < 7
        kw = 14*Tzew + 1642;
    elseif 7 <=Tzew && Tzew < 10
        kw = -170/3*Tzew + 6410/3;
    elseif 10 <=Tzew && Tzew < 20
        kw = -31*Tzew + 1880;
    elseif 20 <=Tzew && Tzew <= 30
        kw = 40*Tzew + 460;
    else
%             fprintf('Error: Tzew out of range [-20;30]\n'); 
        fprintf('Error: Tzew out of range [-15;30]\n'); 
    end
end

== matlab function sim_instalacja_podlogowa_regulacja_pogodowa/qk - pompa ciepła ==
  data: Tzew input; qk output; Twyj input
function qk = fcn(Tzew, Twyj)
qk = 0;
if Twyj >= 50
    if -15 <=Tzew && Tzew < -7
        qk = 445*Tzew + 9995;
    elseif -7 <=Tzew && Tzew < 2
        qk = 830/9*Tzew + 67730/9;
    elseif 2 <=Tzew && Tzew < 7
        qk = 392*Tzew + 6926;
    elseif 7 <=Tzew && Tzew < 10
        qk = -130/3*Tzew + 29920/3;
    elseif 10 <=Tzew && Tzew < 20
        qk = 38*Tzew + 9160;
    elseif 20 <=Tzew && Tzew <= 30
        qk = -56*Tzew + 11040;
    else
         fprintf('Error: Tzew out of range [-15;30]\n'); 
    end
elseif Twyj >= 40 && Twyj < 50
%     if -20 <=Tzew && Tzew < -15
%         qk = 256*Tzew + 9750;
%     elseif -15 <=Tzew && Tzew < 7
    if -15 <=Tzew && Tzew < -7
        qk = 120*Tzew + 7710;
    elseif -7 <=Tzew && Tzew < 2
        qk = 340/3*Tzew + 22990/3;
    elseif 2 <=Tzew && Tzew < 7
        qk = 114*Tzew + 7662;
    elseif 7 <=Tzew && Tzew < 10
        qk = 520/3*Tzew + 21740/3;
    elseif 10 <=Tzew && Tzew < 20
        qk = 16*Tzew + 8820;
    elseif 20 <=Tzew && Tzew <= 30
        qk = -113*Tzew + 11400;
    else
%         fprintf('Error: Tzew out of range [-20;30]\n'); 
        fprintf('Error: Tzew out of range [-15;30]\n'); 
    end
    elseif Twyj < 40
%         if -20 <=Tzew && Tzew < -15
%             qk = 262*Tzew + 10220;
%         elseif -15 <=Tzew && Tzew < -7
        if -15 <=Tzew && Tzew < -7
            qk = -145/4*Tzew + 22985/4;
        elseif -7 <=Tzew && Tzew < 2
            qk = 6000;
        elseif 2 <=Tzew && Tzew < 7
            qk = 426*Tzew + 5148;
        elseif 7 <=Tzew && Tzew < 10
            qk = -190/3*Tzew + 25720/3;
        elseif 10 <=Tzew && Tzew < 20
            qk = 34*Tzew + 7600;
        elseif 20 <=Tzew && Tzew <= 30
            qk = 163*Tzew + 5020;
        else
%             fprintf('Error: Tzew out of range [-20;30]\n'); 
            fprintf('Error: Tzew out of range [-15;30]\n'); 
        end
end

== matlab function sim_instalacja_podlogowa_regulacja_pogodowa/COP ==
  data: Tzew input; COP output; Twyj input
function COP = fcn(Tzew, Twyj)
COP = 0;
if Twyj >= 50
    if -15 <=Tzew && Tzew < -7
        COP = 0.105*Tzew + 2.465;
    elseif -7 <=Tzew && Tzew < 2
        COP = 0.0233*Tzew + 1.89333;
    elseif 2 <=Tzew && Tzew < 7
        COP = 0.148*Tzew + 1.644;
    elseif 7 <=Tzew && Tzew < 10
        COP = 0.05*Tzew + 2.33;
    elseif 10 <=Tzew && Tzew < 20
        COP = 0.006*Tzew + 2.77;
    elseif 20 <=Tzew && Tzew <= 30
        COP = 0.042*Tzew + 2.05;
    else
         fprintf('Error: Tzew out of range [-15;30]\n'); 
    end
elseif Twyj >= 40 && Twyj < 50
%     if -20 <=Tzew && Tzew < -15
%         COP = 0.052*Tzew + 2.62;
%     elseif -15 <=Tzew && Tzew < 7
    if -15 <=Tzew && Tzew < -7
        COP = 0.055*Tzew + 2.665;
    elseif -7 <=Tzew && Tzew < 2
        COP = 0.1*Tzew + 2.98;
    elseif 2 <=Tzew && Tzew < 7
        COP = 0.046*Tzew + 3.088;
    elseif 7 <=Tzew && Tzew < 10
        COP = 0.07*Tzew + 2.92;
    elseif 10 <=Tzew && Tzew < 20
        COP = 0.061*Tzew + 3.01;
    elseif 20 <=Tzew && Tzew <= 30
        COP = 0.051*Tzew + 3.21;
    else
%         fprintf('Error: Tzew out of range [-20;30]\n'); 
        fprintf('Error: Tzew out of range [-15;30]\n'); 
    end
    elseif Twyj < 40
%         if -20 <=Tzew && Tzew < -15
%             COP = 0.064*Tzew + 3.18;
%         elseif -15 <=Tzew && Tzew < -7
        if -15 <=Tzew && Tzew < -7
            COP = 0.06*Tzew + 3.12;
        elseif -7 <=Tzew && Tzew < 2
            COP = 0.1*Tzew + 3.4;
        elseif 2 <=Tzew && Tzew < 7
            COP = 0.212*Tzew + 3.176;
        elseif 7 <=Tzew && Tzew < 10
            COP = 0.11*Tzew + 3.89;
        elseif 10 <=Tzew && Tzew < 20
            COP = 0.158*Tzew + 3.41;
        elseif 20 <=Tzew && Tzew <= 30
            COP = -0.058*Tzew + 7.73;
        else
%             fprintf('Error: Tzew out of range [-20;30]\n'); 
            fprintf('Error: Tzew out of range [-15;30]\n'); 
        end
end

== matlab function sim_instalacja_podlogowa_regulacja_pogodowa/ograniczenie mocy ==
  data: moc input; qk output; Tzew input
function qk = fcn(moc, Tzew)
qk = moc;
if Tzew < -2 
    % wg EN 14511 (A–7/W35)
    if moc < 2700
        qk = 2700;
    elseif moc > 7500
        qk = 7500;
    else
        qk = moc;
    end
elseif Tzew >= -2 && Tzew <= 5
    % wg EN 14511 (A2/W35)
    if moc < 3600
        qk = 3600;
    elseif moc > 9000
        qk = 9000;
    else
        qk = moc;
    end
else
    % wg EN 14511 (A7/W35)
    if moc < 4700
        qk = 4700;
    elseif moc > 12000
        qk = 12000;
    else
        qk = moc;
    end
end

== matlab function sim_instalacja_podlogowa_regulacja_pogodowa/grzałka wspomagajaca ==
  data: Tzew input; q_grz output
function q_grz = fcn(Tzew)
q_grz = 0;
if Tzew <= -9 % punkt biwalentny
    q_grz = 3000;
elseif Tzew > -9 && Tzew <= -8
    q_grz = 2000;
elseif Tzew > -8 && Tzew <= -7
    q_grz = 1500;
elseif Tzew > -7 && Tzew <= -6
    q_grz = 1000;
else
    q_grz = 0;
end

== matlab function sim_instalacja_podlogowa_regulacja_pogodowa/zawor bypass ==
  data: fmb input; fmg input; f_bypass output
function f_bypass = fcn(fmb, fmg)
if fmb + fmg < 0.194 %f min
    f_bypass = 0.194 -fmg - fmb;
else
    f_bypass = 0;
end

== matlab function sim_instalacja_podlogowa_regulacja_pogodowa/przebiegi czasowe zima ==
  data: time input; Tzew output; Tzadana_wew output; Tzadana_cwu output; ogrzewanie_domu output; qt output; qtb output
function [Tzew, Tzadana_wew, Tzadana_cwu, ogrzewanie_domu, qt, qtb] = fcn(time)
Tzew = -4;
Tzadana_wew = 18;
Tzadana_cwu = 41;
ogrzewanie_domu = 1;
qt = 0;
qtb = 0;
if time < 1003600 %6)
    Tzew = -4;
    Tzadana_wew = 20;
    Tzadana_cwu = 41;
    ogrzewanie_domu = 1;
    qt = 0;
    qtb = 0;
elseif 1003600 <= time && time <1007200 %<6;7)
    Tzew = -4;
    Tzadana_wew = 22;
    Tzadana_cwu = 41;
    ogrzewanie_domu = 1;
    qt = 0;
    qtb = -1000;
elseif 1007200 <= time && time <1010800 %<7;8)
    Tzew = -4;
    Tzadana_wew = 22;
    Tzadana_cwu = 41;
    ogrzewanie_domu = 1;
    qt = -1000;
    qtb = -1000;
elseif 1010800 <= time && time <1014400 %<8;9)
    Tzew = -4;
    Tzadana_wew = 20;
    Tzadana_cwu = 41;
    ogrzewanie_domu = 1;
    qt = 0;
    qtb = 0;
elseif 1014400 <= time && time <1025200 %<9;12)
    Tzew = -3;
    Tzadana_wew = 20;
    Tzadana_cwu = 45;
    ogrzewanie_domu = 0;
    qt = 0;
    qtb = 0;
elseif 1025200 <= time && time <1032400 %<12;14)
    Tzew = -2;
    Tzadana_wew = 20;
    Tzadana_cwu = 45;
    ogrzewanie_domu = 0;
    qt = 0;
    qtb = 0;
elseif 1032400 <= time && time <1036000 %<14;15)
    Tzew = -2;
    Tzadana_wew = 20;
    Tzadana_cwu = 45;
    ogrzewanie_domu = 1;
    qt = 0;
    qtb = 0;
elseif 1036000 <= time && time <1039600 %<15;16)
    Tzew = -2;
    Tzadana_wew = 24;
    Tzadana_cwu = 41;
    ogrzewanie_domu = 1;
    qt = 0;
    qtb = 0;
elseif 1039600 <= time && time <1043200 %<16;17)
    Tzew = -2;
    Tzadana_wew = 24;
    Tzadana_cwu = 41;
    ogrzewanie_domu = 1;
    qt = 1000;
    qtb = -1000;
elseif 1043200 <= time && time <1050400 %<17;19)
    Tzew = -3;
    Tzadana_wew = 24;
    Tzadana_cwu = 41;
    ogrzewanie_domu = 1;
    qt = 0;
    qtb = 0;
elseif 1050400 <= time && time <1052200 %<19;19:30)
    Tzew = -4;
    Tzadana_wew = 22;
    Tzadana_cwu = 45;
    ogrzewanie_domu = 1;
    qt = 0;
    qtb = 0;
elseif 1052200 <= time && time <1054000 %<19:30;20)
    Tzew = -4;
    Tzadana_wew = 22;
    Tzadana_cwu = 45;
    ogrzewanie_domu = 1;
    qt = 0;
    qtb = 0;
elseif 1054000 <= time && time <1055800 %<20;20:30)
    Tzew = -4;
    Tzadana_wew = 22;
    Tzadana_cwu = 45;
    ogrzewanie_domu = 0;
    qt = 0;
    qtb = -1000;
elseif 1055800 <= time && time <1057600 %<20:30;21)
    Tzew = -4;
    Tzadana_wew = 22;
    Tzadana_cwu = 45;
    ogrzewanie_domu = 0;
    qt = 0;
    qtb = -1000;
elseif 1057600 <= time && time <1064800 %<21;23)
    Tzew = -6;
    Tzadana_wew = 20;
    Tzadana_cwu = 45;
    ogrzewanie_domu = 1;
    qt = 0;
    qtb = 0;
elseif 1064800 <= time && time <1072000 %<23;1)
    Tzew = -10;
    Tzadana_wew = 18;
    Tzadana_cwu = 45;
    ogrzewanie_domu = 1;
    qt = 0;
    qtb = 0;
elseif 1072000 <= time && time <1079200 %<1;3)
    Tzew = -8;
    Tzadana_wew = 18;
    Tzadana_cwu = 45;
    ogrzewanie_domu = 0;
    qt = 0;
    qtb = 0;
elseif 1079200 <= time && time <1082800 %<3;4)
    Tzew = -6;
    Tzadana_wew = 18;
    Tzadana_cwu = 45;
    ogrzewanie_domu = 0;
    qt = 0;
    qtb = 0;
elseif 1082800 <= time && time <1086400 %<4;5)
    Tzew = -6;
    Tzadana_wew = 18;
    Tzadana_cwu = 45;
    ogrzewanie_domu = 1;
    qt = 0;
    qtb = 0;
elseif 1086400 <= time && time <1100000 %<5;6)
    Tzew = -6;
    Tzadana_wew = 22;
    Tzadana_cwu = 45;
    ogrzewanie_domu = 1;
    qt = 0;
    qtb = 0;
end
